simulink model "exampleNB"  (Simulink 8.0)
settings: Solver=ode45  StartTime=0.0  StopTime=10.0  RelTol=1e-3
values from neighbouring files (symbols this model uses):
  f = logspace(1,3,1e3)    [run_NB.m]
undefined symbols (not defined in the file or in its folder): exampleOpt, OptickleFlexTF
libraries: NbLibrary x10, cstblocks x1
settings Model: Creator=nicolas  LastModifiedBy=ccw
settings DataIOCC: SignalLoggingSaveFormat=ModelDataLogs
settings DebuggingCC: FcnCallInpInsideContextMsg=EnableAllAsWarning  FrameProcessingCompatibilityMsg=error
settings CodeAppCC: CustomSymbolStrType=$N$R$M_T
settings GRTTargetCC: CodeReplacementLibrary=C89/C90 (ANSI)

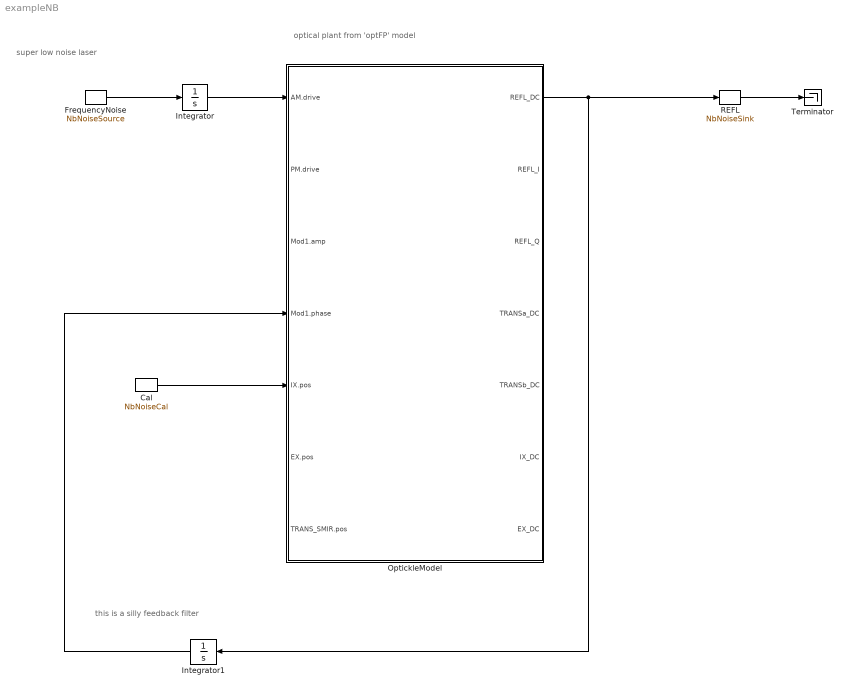
== system exampleNB ==
  note: optical plant from 'optFP' model
  note: this is a silly feedback filter
  note: super low noise laser
  Cal : NbLibrary/NbNoiseCal  Tag=NbNoiseCal  dof='REFLI'  unit='m/rt(Hz)'
      settings: AttributesFormatString=%<Tag>
  FrequencyNoise : NbLibrary/NbNoiseSource  Tag=NbNoiseSource  asd=1e-7  chan=''  groupNest=1  group='Laser Frequency'  subgroup=''  subsubgroup=''  subsubsubgroup=''
      settings: AttributesFormatString=%<Tag>
  Integrator : Integrator
  Integrator1 : Integrator
  OptickleModel : Subsystem  Description=Autogenerated using OptickleFlexTF.buildSys('exampleOpt','f','00')
      settings: AttributesFormatString=%<Description>
  REFL : NbLibrary/NbNoiseSink  Tag=NbNoiseSink  dof='REFLI'  asd=''  chan=''
      settings: AttributesFormatString=%<Tag>
  Terminator : Terminator
  wires:
  Cal/1 -> OptickleModel/5(IX.pos)
  FrequencyNoise/1 -> Integrator/1
  OptickleModel/1(REFL_DC) -> Integrator1/1, REFL/1
  Integrator/1 -> OptickleModel/1(AM.drive)
  Integrator1/1 -> OptickleModel/4(Mod1.phase)
  REFL/1 -> Terminator/1

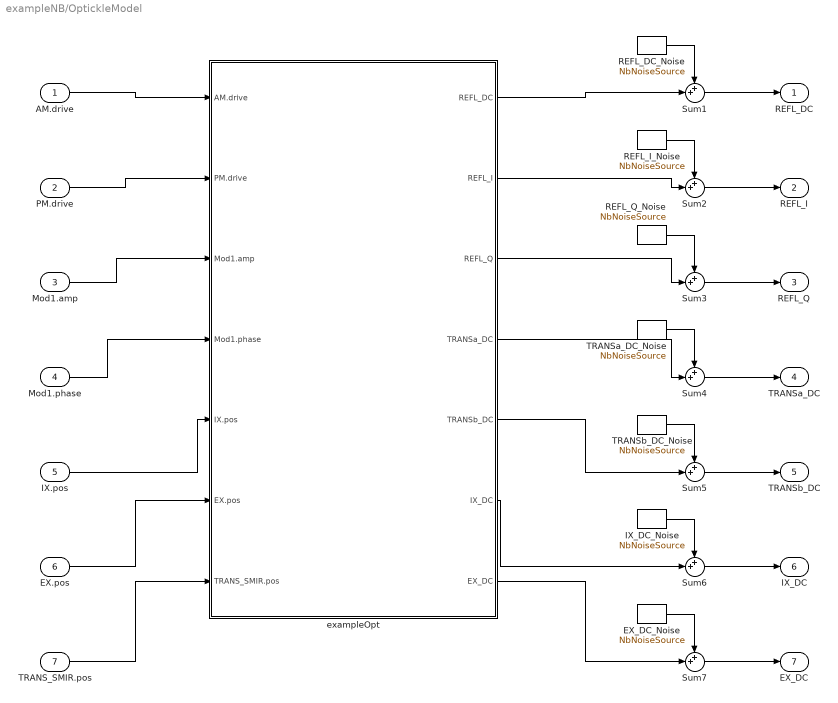
== system exampleNB/OptickleModel ==
  AM.drive : Inport
  PM.drive : Inport  Port=2
  Mod1.amp : Inport  Port=3
  Mod1.phase : Inport  Port=4
  IX.pos : Inport  Port=5
  EX.pos : Inport  Port=6
  TRANS_SMIR.pos : Inport  Port=7
  EX_DC_Noise : NbLibrary/NbNoiseSource  Tag=NbNoiseSource  asd=OptickleFlexTF.noiseBlock(exampleOpt,f,'00','EX_DC',OptickleFlexTF.makeDriveIndex(exampleOpt,{'AM.drive','PM.drive','Mod1.amp','Mod1.phase','IX.pos','EX.pos','TRANS_SMIR.pos'}))  chan=''  groupNest=2  group='Quantum Vacuum'  subgroup='EX_DC'  subsubgroup=''  subsubsubgroup=''
      settings: AttributesFormatString=%<Tag>
  IX_DC_Noise : NbLibrary/NbNoiseSource  Tag=NbNoiseSource  asd=OptickleFlexTF.noiseBlock(exampleOpt,f,'00','IX_DC',OptickleFlexTF.makeDriveIndex(exampleOpt,{'AM.drive','PM.drive','Mod1.amp','Mod1.phase','IX.pos','EX.pos','TRANS_SMIR.pos'}))  chan=''  groupNest=2  group='Quantum Vacuum'  subgroup='IX_DC'  subsubgroup=''  subsubsubgroup=''
      settings: AttributesFormatString=%<Tag>
  REFL_DC_Noise : NbLibrary/NbNoiseSource  Tag=NbNoiseSource  asd=OptickleFlexTF.noiseBlock(exampleOpt,f,'00','REFL_DC',OptickleFlexTF.makeDriveIndex(exampleOpt,{'AM.drive','PM.drive','Mod1.amp','Mod1.phase','IX.pos','EX.pos','TRANS_SMIR.pos'}))  chan=''  groupNest=2  group='Quantum Vacuum'  subgroup='REFL_DC'  subsubgroup=''  subsubsubgroup=''
      settings: AttributesFormatString=%<Tag>
  REFL_I_Noise : NbLibrary/NbNoiseSource  Tag=NbNoiseSource  asd=OptickleFlexTF.noiseBlock(exampleOpt,f,'00','REFL_I',OptickleFlexTF.makeDriveIndex(exampleOpt,{'AM.drive','PM.drive','Mod1.amp','Mod1.phase','IX.pos','EX.pos','TRANS_SMIR.pos'}))  chan=''  groupNest=2  group='Quantum Vacuum'  subgroup='REFL_I'  subsubgroup=''  subsubsubgroup=''
      settings: AttributesFormatString=%<Tag>
  REFL_Q_Noise : NbLibrary/NbNoiseSource  Tag=NbNoiseSource  asd=OptickleFlexTF.noiseBlock(exampleOpt,f,'00','REFL_Q',OptickleFlexTF.makeDriveIndex(exampleOpt,{'AM.drive','PM.drive','Mod1.amp','Mod1.phase','IX.pos','EX.pos','TRANS_SMIR.pos'}))  chan=''  groupNest=2  group='Quantum Vacuum'  subgroup='REFL_Q'  subsubgroup=''  subsubsubgroup=''
      settings: AttributesFormatString=%<Tag>
  Sum{1..7} (7 alike) : Sum  Inputs=++|  SaturateOnIntegerOverflow=on  InputSameDT=on  OutDataTypeStr=Inherit: Same as first input
  TRANSa_DC_Noise : NbLibrary/NbNoiseSource  Tag=NbNoiseSource  asd=OptickleFlexTF.noiseBlock(exampleOpt,f,'00','TRANSa_DC',OptickleFlexTF.makeDriveIndex(exampleOpt,{'AM.drive','PM.drive','Mod1.amp','Mod1.phase','IX.pos','EX.pos','TRANS_SMIR.pos'}))  chan=''  groupNest=2  group='Quantum Vacuum'  subgroup='TRANSa_DC'  subsubgroup=''  subsubsubgroup=''
      settings: AttributesFormatString=%<Tag>
  TRANSb_DC_Noise : NbLibrary/NbNoiseSource  Tag=NbNoiseSource  asd=OptickleFlexTF.noiseBlock(exampleOpt,f,'00','TRANSb_DC',OptickleFlexTF.makeDriveIndex(exampleOpt,{'AM.drive','PM.drive','Mod1.amp','Mod1.phase','IX.pos','EX.pos','TRANS_SMIR.pos'}))  chan=''  groupNest=2  group='Quantum Vacuum'  subgroup='TRANSb_DC'  subsubgroup=''  subsubsubgroup=''
      settings: AttributesFormatString=%<Tag>
  exampleOpt : Subsystem  Description=OptickleFlexTF(exampleOpt,f,'00',{'AM.drive','PM.drive','Mod1.amp','Mod1.phase','IX.pos','EX.pos','TRANS_SMIR.pos'},{'REFL_DC','REFL_I','REFL_Q','TRANSa_DC','TRANSb_DC','IX_DC','EX_DC'})  SCDEnableBlockLinearizationSpecification=on
      settings: AttributesFormatString=%<Description>
  REFL_DC : Outport
  REFL_I : Outport  Port=2
  REFL_Q : Outport  Port=3
  TRANSa_DC : Outport  Port=4
  TRANSb_DC : Outport  Port=5
  IX_DC : Outport  Port=6
  EX_DC : Outport  Port=7
  wires:
  AM.drive/1 -> exampleOpt/1(AM.drive)
  PM.drive/1 -> exampleOpt/2(PM.drive)
  Mod1.amp/1 -> exampleOpt/3(Mod1.amp)
  Mod1.phase/1 -> exampleOpt/4(Mod1.phase)
  IX.pos/1 -> exampleOpt/5(IX.pos)
  EX.pos/1 -> exampleOpt/6(EX.pos)
  TRANS_SMIR.pos/1 -> exampleOpt/7(TRANS_SMIR.pos)
  REFL_DC_Noise/1 -> Sum1/1
  exampleOpt/1(REFL_DC) -> Sum1/2
  Sum1/1 -> REFL_DC/1
  REFL_I_Noise/1 -> Sum2/1
  exampleOpt/2(REFL_I) -> Sum2/2
  Sum2/1 -> REFL_I/1
  REFL_Q_Noise/1 -> Sum3/1
  exampleOpt/3(REFL_Q) -> Sum3/2
  Sum3/1 -> REFL_Q/1
  TRANSa_DC_Noise/1 -> Sum4/1
  exampleOpt/4(TRANSa_DC) -> Sum4/2
  Sum4/1 -> TRANSa_DC/1
  TRANSb_DC_Noise/1 -> Sum5/1
  exampleOpt/5(TRANSb_DC) -> Sum5/2
  Sum5/1 -> TRANSb_DC/1
  IX_DC_Noise/1 -> Sum6/1
  exampleOpt/6(IX_DC) -> Sum6/2
  Sum6/1 -> IX_DC/1
  EX_DC_Noise/1 -> Sum7/1
  exampleOpt/7(EX_DC) -> Sum7/2
  Sum7/1 -> EX_DC/1

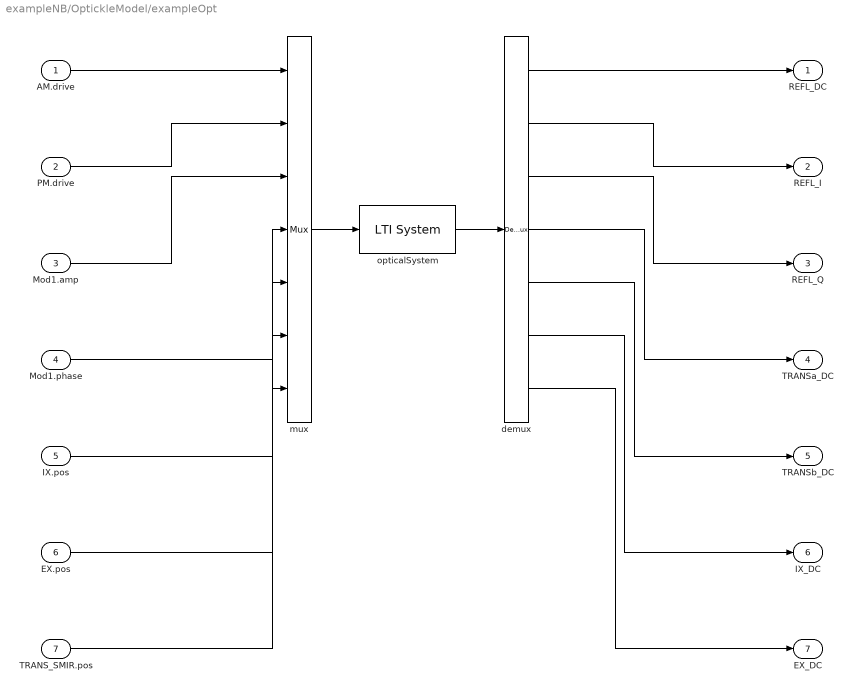
== system exampleNB/OptickleModel/exampleOpt ==
  AM.drive : Inport
  PM.drive : Inport  Port=2
  Mod1.amp : Inport  Port=3
  Mod1.phase : Inport  Port=4
  IX.pos : Inport  Port=5
  EX.pos : Inport  Port=6
  TRANS_SMIR.pos : Inport  Port=7
  demux : Demux  Outputs=7
  mux : Mux  Inputs=7
  opticalSystem : cstblocks/LTI System  sys=repmat(tf(1),[7,7])  IC=[]
  REFL_DC : Outport
  REFL_I : Outport  Port=2
  REFL_Q : Outport  Port=3
  TRANSa_DC : Outport  Port=4
  TRANSb_DC : Outport  Port=5
  IX_DC : Outport  Port=6
  EX_DC : Outport  Port=7
  wires:
  mux/1 -> opticalSystem/1
  opticalSystem/1 -> demux/1
  AM.drive/1 -> mux/1
  PM.drive/1 -> mux/2
  Mod1.amp/1 -> mux/3
  Mod1.phase/1 -> mux/4
  IX.pos/1 -> mux/5
  EX.pos/1 -> mux/6
  TRANS_SMIR.pos/1 -> mux/7
  demux/1 -> REFL_DC/1
  demux/2 -> REFL_I/1
  demux/3 -> REFL_Q/1
  demux/4 -> TRANSa_DC/1
  demux/5 -> TRANSb_DC/1
  demux/6 -> IX_DC/1
  demux/7 -> EX_DC/1
